simulink model "Liver"  (R2019a)
settings: Solver=VariableStepAuto  StartTime=0.0  StopTime=10.0  RelTol=1e-3
undefined symbols (not defined in the file): Q_gA, Q_gG, Q_gL, V_gK, V_gL
settings Model: Creator=jcp2  LastModifiedBy=rache

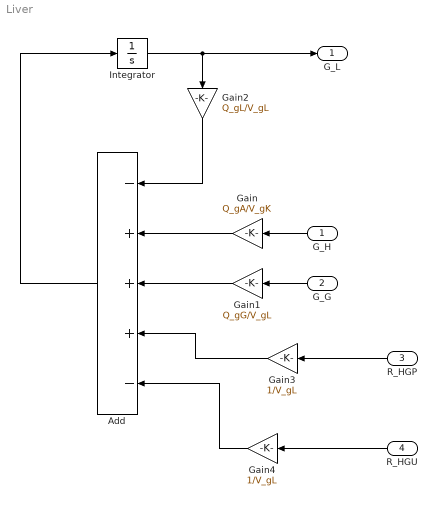
== system Liver ==
  G_H : Inport
  G_G : Inport  Port=2
  R_HGP : Inport  Port=3
  R_HGU : Inport  Port=4
  Add : Sum  Inputs=-+++-
  Gain : Gain  Gain=Q_gA/V_gK
  Gain1 : Gain  Gain=Q_gG/V_gL
  Gain2 : Gain  Gain=Q_gL/V_gL
  Gain3 : Gain  Gain=1/V_gL
  Gain4 : Gain  Gain=1/V_gL
  Integrator : Integrator
  G_L : Outport
  wires:
  Integrator/1 -> Gain2/1, G_L/1
  G_G/1 -> Gain1/1
  G_H/1 -> Gain/1
  Gain4/1 -> Add/5
  Gain3/1 -> Add/4
  Gain1/1 -> Add/3
  Gain/1 -> Add/2
  Gain2/1 -> Add/1
  Add/1 -> Integrator/1
  R_HGP/1 -> Gain3/1
  R_HGU/1 -> Gain4/1
